simulink model "sampleIT"  (R2018a)
settings: Solver=VariableStepAuto  StartTime=0.0  StopTime=10.0  RelTol=1e-3
settings Model: Creator=mattclark  LastModifiedBy=mattclark
settings SFSimCC: SimUserSources=doubleIT.c  SimUserLibraries=monitor.o
settings SFSimCC: SimCustomHeaderCode=|
  | #include "doubleIT.h"
  | #include "monitor.h"

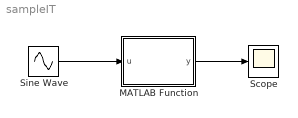
== system sampleIT ==
  MATLAB Function : MATLAB Function  TreatAsAtomicUnit=on
  Scope : Scope
  Sine Wave : Sin  Amplitude=100  SampleTime=0
  wires:
  Sine Wave/1 -> MATLAB Function/1(u)
  MATLAB Function/1(y) -> Scope/1

== matlab function sampleIT/MATLAB Function ==
  data: u input; y output
function y = driver(u)
y = 0.0;
y = coder.ceval('sampleIT',u);
